simulink model "two_tanks_model_PI"  (R2018b)
settings: Solver=FixedStepAuto  StartTime=0.0  StopTime=600  FixedStep=0.1  RelTol=1e-3
model workspace (MATLAB code in the model file):
  | A1 = 1;
  | a1 = 0.1*0.1;
  | A2 = A1;
  | a2 = a1;
  | h10 = 1;
  | h20=1;
libraries: simulink x1
settings Model: PacingRate=10  Creator=kjartan  LastModifiedBy=kjartan

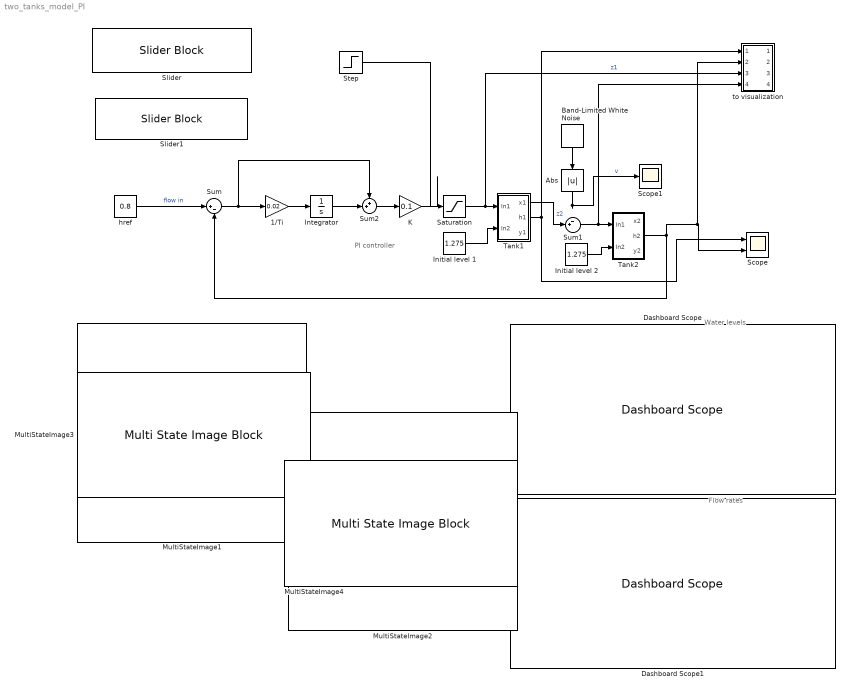
== system two_tanks_model_PI ==
  note: Flow rates
  note: PI controller
  note: Water levels
  1/Ti : Gain  Gain=0.02
  Abs : Abs
  Band-Limited White Noise : simulink/Sources/Band-Limited White Noise  Cov=0.01*0.01  Ts=3  seed=[23341]
  Dashboard Scope : DashboardScope  WebBlockId=50  Ymin=0  Ymax=2.6000000000000001
  Dashboard Scope1 : DashboardScope  WebBlockId=91  Ymin=0  Ymax=0.29999999999999999
  Initial level 1 : Constant  Value=1.275
  Initial level 2 : Constant  Value=1.275
  Integrator : Integrator
  K : Gain  Gain=0.1
  MultiStateImage1 : MultiStateImageBlock  WebBlockId=71
  MultiStateImage2 : MultiStateImageBlock  WebBlockId=119
  MultiStateImage3 : MultiStateImageBlock  WebBlockId=117  ScaleMode=Fill
  MultiStateImage4 : MultiStateImageBlock  WebBlockId=126  ScaleMode=Fill
  Saturation : Saturate  LowerLimit=0
  Scope : Scope  NumInputPorts=2
  Scope1 : Scope
  Slider : SliderBlock  WebBlockId=82  ScaleMax=0.5
  Slider1 : SliderBlock  WebBlockId=85  ScaleMax=0.059999999999999998
  Step : Step  Time=100  Before=0.05  After=0.65  SampleTime=0
  Sum : Sum  Inputs=|+-
  Sum1 : Sum  Inputs=-+|
  Sum2 : Sum  Inputs=++|
  Tank1 : Subsystem
  Tank2 : Subsystem
  href : Constant  Value=0.8
  to visualization : Subsystem
  wires:
  Tank1/1(x1) -> Sum1/2  "z2"
  Tank1/2(h1) -> to visualization/1(In2), Scope/1
  Tank2/2(h2) -> to visualization/2(In1), Scope/2, Sum/2
  Sum1/1 -> to visualization/4(In4), Tank2/1(In1)
  Band-Limited White Noise/1 -> Abs/1
  Abs/1 -> Scope1/1  "v"
  href/1 -> Sum/1  "flow in"
  Integrator/1 -> Sum2/2
  Sum/1 -> Sum2/1, 1/Ti/1
  Sum2/1 -> K/1
  1/Ti/1 -> Integrator/1
  Saturation/1 -> to visualization/3(In3), Tank1/1(In1)  "z1"
  K/1 -> ?
  Initial level 2/1 -> Tank2/2(In2)
  Initial level 1/1 -> Tank1/2(In2)
  Step/1 -> Saturation/1

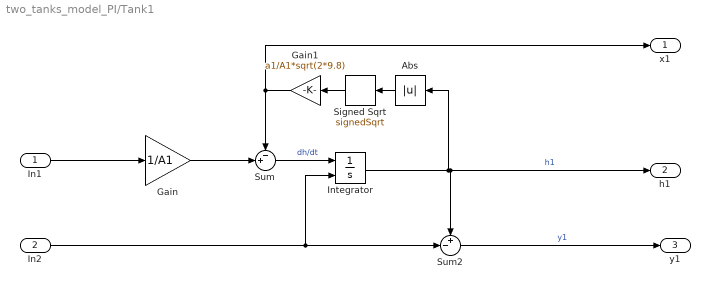
== system two_tanks_model_PI/Tank1 ==
  In1 : Inport
  In2 : Inport  Port=2
  Abs : Abs
  Gain : Gain  Gain=1/A1
  Gain1 : Gain  Gain=a1/A1*sqrt(2*9.8)
  Integrator : Integrator  InitialConditionSource=external  InitialCondition=h10
  Signed Sqrt : Sqrt  Operator=signedSqrt  SaturateOnIntegerOverflow=on
  Sum : Sum  Inputs=-+|
  Sum2 : Sum  Inputs=+-|
  x1 : Outport
  h1 : Outport  Port=2
  y1 : Outport  Port=3
  wires:
  Gain1/1 -> x1/1, Sum/1
  Gain/1 -> Sum/2
  Sum/1 -> Integrator/1  "dh/dt"
  In1/1 -> Gain/1
  Sum2/1 -> y1/1  "y1"
  Signed Sqrt/1 -> Gain1/1
  Integrator/1 -> h1/1, Sum2/1, Abs/1  "h1"
  Abs/1 -> Signed Sqrt/1
  In2/1 -> Sum2/2, Integrator/2

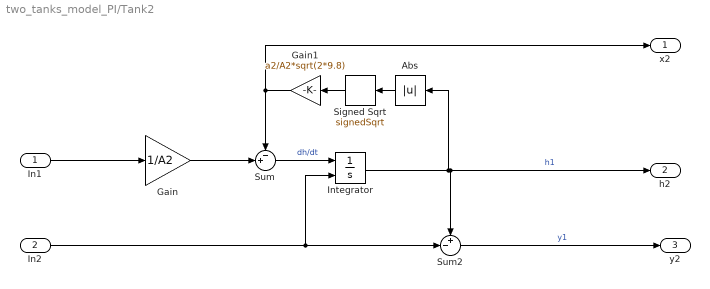
== system two_tanks_model_PI/Tank2 ==
  In1 : Inport
  In2 : Inport  Port=2
  Abs : Abs
  Gain : Gain  Gain=1/A2
  Gain1 : Gain  Gain=a2/A2*sqrt(2*9.8)
  Integrator : Integrator  InitialConditionSource=external  InitialCondition=h10
  Signed Sqrt : Sqrt  Operator=signedSqrt  SaturateOnIntegerOverflow=on
  Sum : Sum  Inputs=-+|
  Sum2 : Sum  Inputs=+-|
  x2 : Outport
  h2 : Outport  Port=2
  y2 : Outport  Port=3
  wires:
  Gain1/1 -> x2/1, Sum/1
  Gain/1 -> Sum/2
  Sum/1 -> Integrator/1  "dh/dt"
  In1/1 -> Gain/1
  Sum2/1 -> y2/1  "y1"
  Signed Sqrt/1 -> Gain1/1
  Integrator/1 -> h2/1, Sum2/1, Abs/1  "h1"
  Abs/1 -> Signed Sqrt/1
  In2/1 -> Sum2/2, Integrator/2

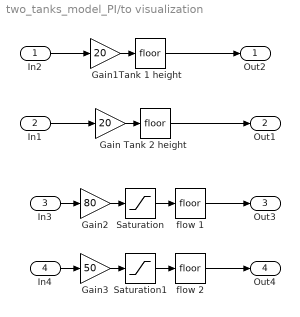
== system two_tanks_model_PI/to visualization ==
  In2 : Inport
  In1 : Inport  Port=2
  In3 : Inport  Port=3
  In4 : Inport  Port=4
  Gain : Gain  Gain=20
  Gain1 : Gain  Gain=20
  Gain2 : Gain  Gain=80
  Gain3 : Gain  Gain=50
  Saturation : Saturate  UpperLimit=10  LowerLimit=0
  Saturation1 : Saturate  UpperLimit=5  LowerLimit=0
  Tank 1 height : Rounding
  Tank 2 height : Rounding
  flow 1 : Rounding
  flow 2 : Rounding
  Out2 : Outport
  Out1 : Outport  Port=2
  Out3 : Outport  Port=3
  Out4 : Outport  Port=4
  wires:
  Tank 2 height/1 -> Out1/1
  Gain/1 -> Tank 2 height/1
  In1/1 -> Gain/1
  Tank 1 height/1 -> Out2/1
  Gain1/1 -> Tank 1 height/1
  In2/1 -> Gain1/1
  flow 1/1 -> Out3/1
  Gain2/1 -> Saturation/1
  In3/1 -> Gain2/1
  flow 2/1 -> Out4/1
  In4/1 -> Gain3/1
  Gain3/1 -> Saturation1/1
  Saturation/1 -> flow 1/1
  Saturation1/1 -> flow 2/1
